simulink model "Ex7_2"  (Simulink 6.0)
settings: Solver=FixedStepDiscrete  SolverMode=SingleTasking  StartTime=0.0  StopTime=Ts*10  FixedStep=Ts  RelTol=1e-3  AbsTol=1e-6
values from neighbouring files (symbols this model uses):
  Ampl = 10^(Amp_dB/20)-pi/1024    (= 0.498119272052)    [Ex7_2Launch.m]
  ClipDAC = (levelsDAC-1)*DeltaDAC/2    (= 22.7142857143)    [Ex7_2Launch.m]
  finrad = Fin*2*pi    (= 136379.482335)    [Ex7_2Launch.m]
  MultiBit = 0    [Ex7_2Launch.m]
  Ncomp = 7    [Ex7_2Launch.m]
  Ts = 1/Fs    (= 3.54308390023e-07)    [Ex7_2Launch.m]
  VrefN = -1    [Ex7_2Launch.m]
  VrefP = 1    [Ex7_2Launch.m]
undefined symbols (not defined in the file or in its folder): Quantiz
settings Model: Creator=francomaloberti  LastModifiedBy=Cri  ExtModeAutoUpdateStatusClock=off
settings DataIOCC: LimitDataPoints=off  SignalLoggingName=sigsOut
settings OptimizationCC: BooleanDataType=off  InlineInvariantSignals=off
settings DebuggingCC: SolverPrmCheckMsg=none
settings HardwareCC: TargetUnknown=on

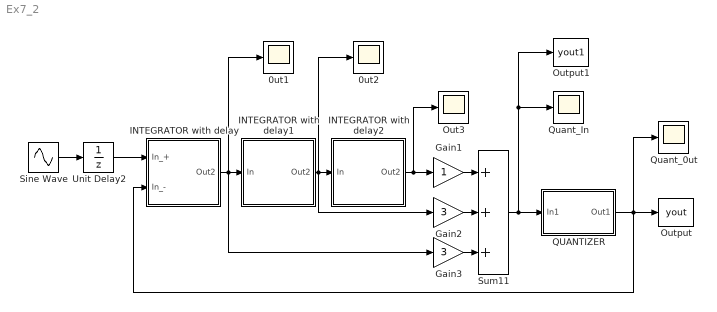
== system Ex7_2 ==
  0ut1 : Scope
  0ut2 : Scope
      settings: TimeRange=0.003  YMin=-1  YMax=1  SaveName=ScopeData2
  Gain1 : Gain
  Gain2 : Gain  Gain=3
  Gain3 : Gain  Gain=3
  INTEGRATOR with delay : Subsystem
      mask Display:
      | patch([10 40 10 10], [0 20 40 0],[1 0 1])
      | plot([10 40 10 10], [0 20 40 0])
      | plot([0 10], [8 8])
      | plot([0 10], [28 28])
      | dpoly([0 1], [1 -1], 'z-')
      | port_label('input', 1, '+')
      | port_label('input', 2, '-')
  INTEGRATOR with delay1 : Subsystem
      mask Display:
      | patch([10 40 10 10], [0 20 40 0],[1 1 0])
      | plot([10 40 10 10], [0 20 40 0])
      | plot([0 10], [20 20])
      | dpoly([0 1], [1 -1], 'z-')
      | port_label('input', 1, 'in')
  INTEGRATOR with delay2 : Subsystem
      mask Display:
      | patch([10 40 10 10], [0 20 40 0],[0 0 1])
      | plot([10 40 10 10], [0 20 40 0])
      | plot([0 10], [20 20])
      | dpoly([0 1], [1 -1], 'z-')
      | port_label('input', 1, 'in')
  Out3 : Scope
      settings: TimeRange=0.003  YMin=-1  YMax=1  SaveName=ScopeData4
  Output : ToWorkspace  VariableName=yout  SampleTime=Ts  SaveFormat=Array
  Output1 : ToWorkspace  VariableName=yout1  SampleTime=Ts  SaveFormat=Array
  QUANTIZER : Subsystem
      mask Display:
      | plot([0 5 5 10 10 15 15], [0 0 5 5 10 10 15])
      | plot([25 30 30 35], [0 0 15 15])
      | disp('  or')
  Quant_0ut : Scope
      settings: TimeRange=0.002937925170068027
  Quant_In : Scope
      settings: TimeRange=0.003  YMin=-1  YMax=1  SaveName=ScopeData3
  Sine Wave : Sin  Amplitude=Ampl  Frequency=finrad  SampleTime=0
  Sum11 : Sum  Inputs=+++  SaturateOnIntegerOverflow=on  InputSameDT=on
  Unit Delay2 : UnitDelay  SampleTime=Ts
  wires:
  Sine Wave/1 -> Unit Delay2/1
  Unit Delay2/1 -> INTEGRATOR with delay/1(In_+)
  INTEGRATOR with delay/1(Out2) -> Gain3/1, 0ut1/1, INTEGRATOR with delay1/1(In)
  INTEGRATOR with delay1/1(Out2) -> 0ut2/1, INTEGRATOR with delay2/1(In), Gain2/1
  Sum11/1 -> Quant_In/1, Output1/1, QUANTIZER/1(In1)
  Gain1/1 -> Sum11/1
  Gain2/1 -> Sum11/2
  Gain3/1 -> Sum11/3
  INTEGRATOR with delay2/1(Out2) -> Gain1/1, Out3/1
  QUANTIZER/1(Out1) -> Output/1, Quant_0ut/1, INTEGRATOR with delay/2(In_-)

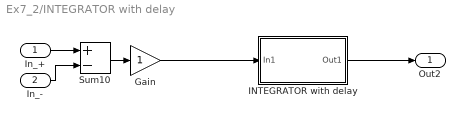
== system Ex7_2/INTEGRATOR with delay ==
  In_+ : Inport  Port=1  LatchInput=off
  In_- : Inport  Port=2  LatchInput=off
  Gain : Gain  SaturateOnIntegerOverflow=on
  INTEGRATOR with delay : Subsystem
      mask Display:
      | patch([0 20 0 0], [0 10 20 0],[0 1 0])
      | text(5,10,'\bf\int','texmode','on')
      | plot([0 20 0 0], [0 10 20 0])
  Sum10 : Sum  Inputs=+-  SaturateOnIntegerOverflow=on  InputSameDT=on
  Out2 : Outport
  wires:
  Gain/1 -> INTEGRATOR with delay/1(In1)
  Sum10/1 -> Gain/1
  In_-/1 -> Sum10/2
  In_+/1 -> Sum10/1
  INTEGRATOR with delay/1(Out1) -> Out2/1

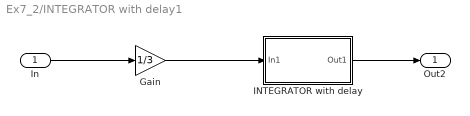
== system Ex7_2/INTEGRATOR with delay1 ==
  In : Inport  Port=1  LatchInput=off
  Gain : Gain  Gain=1/3  SaturateOnIntegerOverflow=on
  INTEGRATOR with delay : Subsystem
      mask Display:
      | patch([0 20 0 0], [0 10 20 0],[0 1 0])
      | text(5,10,'\bf\int','texmode','on')
      | plot([0 20 0 0], [0 10 20 0])
  Out2 : Outport
  wires:
  Gain/1 -> INTEGRATOR with delay/1(In1)
  In/1 -> Gain/1
  INTEGRATOR with delay/1(Out1) -> Out2/1

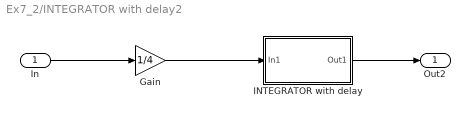
== system Ex7_2/INTEGRATOR with delay2 ==
  In : Inport  Port=1  LatchInput=off
  Gain : Gain  Gain=1/4  SaturateOnIntegerOverflow=on
  INTEGRATOR with delay : Subsystem
      mask Display:
      | patch([0 20 0 0], [0 10 20 0],[0 1 0])
      | text(5,10,'\bf\int','texmode','on')
      | plot([0 20 0 0], [0 10 20 0])
  Out2 : Outport
  wires:
  Gain/1 -> INTEGRATOR with delay/1(In1)
  In/1 -> Gain/1
  INTEGRATOR with delay/1(Out1) -> Out2/1

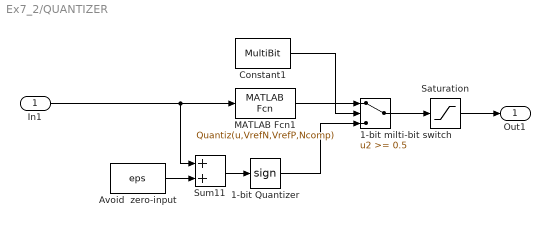
== system Ex7_2/QUANTIZER ==
  In1 : Inport  Port=1  LatchInput=off
  1-bit Quantizer : Signum
  1-bit milti-bit switch : Switch  Threshold=0.5
  Avoid  zero-input : Constant  Value=eps
  Constant1 : Constant  Value=MultiBit
  MATLAB Fcn1 : MATLABFcn  MATLABFcn=Quantiz(u,VrefN,VrefP,Ncomp)
  Saturation : Saturate  UpperLimit=ClipDAC  LowerLimit=-ClipDAC
  Sum11 : Sum  SaturateOnIntegerOverflow=on  InputSameDT=on
  Out1 : Outport
  wires:
  In1/1 -> MATLAB Fcn1/1, Sum11/1
  MATLAB Fcn1/1 -> 1-bit milti-bit switch/1
  1-bit Quantizer/1 -> 1-bit milti-bit switch/3
  Constant1/1 -> 1-bit milti-bit switch/2
  1-bit milti-bit switch/1 -> Saturation/1
  Sum11/1 -> 1-bit Quantizer/1
  Avoid  zero-input/1 -> Sum11/2
  Saturation/1 -> Out1/1

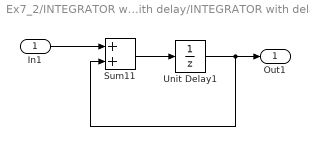
== system Ex7_2/INTEGRATOR with delay/INTEGRATOR with delay ==
  In1 : Inport  Port=1  LatchInput=off
  Sum11 : Sum  SaturateOnIntegerOverflow=on  InputSameDT=on
  Unit Delay1 : UnitDelay  SampleTime=Ts
  Out1 : Outport
  wires:
  In1/1 -> Sum11/1
  Sum11/1 -> Unit Delay1/1
  Unit Delay1/1 -> Out1/1, Sum11/2

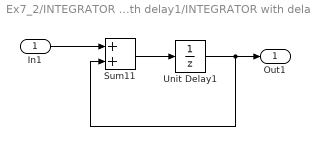
== system Ex7_2/INTEGRATOR with delay1/INTEGRATOR with delay ==
  In1 : Inport  Port=1  LatchInput=off
  Sum11 : Sum  SaturateOnIntegerOverflow=on  InputSameDT=on
  Unit Delay1 : UnitDelay  SampleTime=Ts
  Out1 : Outport
  wires:
  In1/1 -> Sum11/1
  Sum11/1 -> Unit Delay1/1
  Unit Delay1/1 -> Out1/1, Sum11/2

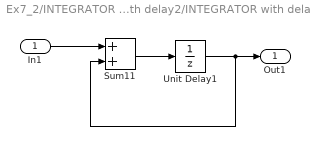
== system Ex7_2/INTEGRATOR with delay2/INTEGRATOR with delay ==
  In1 : Inport  Port=1  LatchInput=off
  Sum11 : Sum  SaturateOnIntegerOverflow=on  InputSameDT=on
  Unit Delay1 : UnitDelay  SampleTime=Ts
  Out1 : Outport
  wires:
  In1/1 -> Sum11/1
  Sum11/1 -> Unit Delay1/1
  Unit Delay1/1 -> Out1/1, Sum11/2
